simulink model "contacto_nuevo"  (Simulink 7.6)
settings: Solver=ode45  StartTime=0.0  StopTime=10.0  FixedStep=0.0001  MaxStep=0.0001  RelTol=1e-3
values from neighbouring files (symbols this model uses):
  b = 5E-5    (= 5e-05)    [Constants.m]
  J = 1    [Constants.m]
  Ke = 1.356    [Constants.m]
undefined symbols (not defined in the file or in its folder): Be, Par_motor, qe
settings Model: Creator=rzotovic  LastModifiedBy=rzotovic  ExtModeTrigMode=oneshot  ExtModeArmWhenConnect=off
settings SolverCC: InitialStep=0.0001
settings DataIOCC: LimitDataPoints=off
settings OptimizationCC: BlockReduction=off  BooleanDataType=off
settings DebuggingCC: SaveWithParameterizedLinksMsg=none  SignalResolutionControl=TryResolveAllWithWarning  SolverPrmCheckMsg=none  MultiTaskDSMMsg=warning  MultiTaskCondExecSysMsg=none  StrictBusMsg=None
settings HardwareCC: TargetUnknown=on
settings RTWCC: IncludeERTFirstTime=on

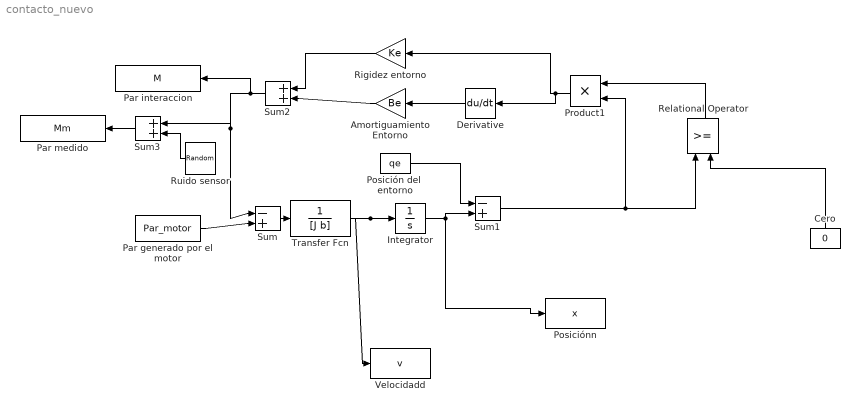
== system contacto_nuevo ==
  Amortiguamiento Entorno : Gain  Gain=Be  SaturateOnIntegerOverflow=on  OutDataTypeStr=Inherit: Same as input  ParamDataTypeStr=Inherit: Same as input
  Cero : Constant  Value=0
  Derivative : Derivative
  Integrator : Integrator
  Par generado por el motor : Constant  Value=Par_motor
  Par interaccion : ToWorkspace  VariableName=M  SampleTime=-1  SaveFormat=Array
  Par medido : ToWorkspace  VariableName=Mm  SampleTime=-1  SaveFormat=Array
  Posición del  entorno : Constant  Value=qe
  Posiciónn : ToWorkspace  VariableName=x  SampleTime=-1  SaveFormat=Array
  Product1 : Product  SaturateOnIntegerOverflow=on  RndMeth=Zero  InputSameDT=on  OutDataTypeStr=Inherit: Same as first input
  Relational Operator : RelationalOperator  InputSameDT=on
  Rigidez entorno : Gain  Gain=Ke  SaturateOnIntegerOverflow=on  OutDataTypeStr=Inherit: Same as input  ParamDataTypeStr=Inherit: Same as input
  Ruido sensor : UniformRandomNumber  Minimum=-0.5  Maximum=0.5  SampleTime=0.1
  Sum : Sum  Inputs=|-+  SaturateOnIntegerOverflow=on  InputSameDT=on  OutDataTypeStr=Inherit: Same as first input
  Sum1 : Sum  Inputs=|-+  SaturateOnIntegerOverflow=on  InputSameDT=on  OutDataTypeStr=Inherit: Same as first input
  Sum2 : Sum  Inputs=|++  SaturateOnIntegerOverflow=on  InputSameDT=on  OutDataTypeStr=Inherit: Same as first input
  Sum3 : Sum  Inputs=|++  SaturateOnIntegerOverflow=on  InputSameDT=on  OutDataTypeStr=Inherit: Same as first input
  Transfer Fcn : TransferFcn  Denominator=[J b]
  Velocidadd : ToWorkspace  VariableName=v  SampleTime=-1  SaveFormat=Array
  wires:
  Par generado por el motor/1 -> Sum/2
  Sum/1 -> Transfer Fcn/1
  Rigidez entorno/1 -> Sum2/1
  Amortiguamiento Entorno/1 -> Sum2/2
  Sum2/1 -> Par interaccion/1, Sum/1, Sum3/1
  Posición del  entorno/1 -> Sum1/1
  Derivative/1 -> Amortiguamiento Entorno/1
  Transfer Fcn/1 -> Integrator/1, Velocidadd/1
  Integrator/1 -> Sum1/2, Posiciónn/1
  Cero/1 -> Relational Operator/2
  Relational Operator/1 -> Product1/1
  Sum1/1 -> Relational Operator/1, Product1/2
  Product1/1 -> Rigidez entorno/1, Derivative/1
  Sum3/1 -> Par medido/1
  Ruido sensor/1 -> Sum3/2
